simulink model "integracion_ikine"  (R2023b)
settings: Solver=FixedStepDiscrete  StartTime=0.0  StopTime=inf  RelTol=1e-3  EnableMultiTasking=on
undefined symbols (not defined in the file): LF
libraries: instrumentseriallib x3, svdutilitieslib x1, dspnetwork x1
settings Model: SimulationMode=accelerator  Creator=gianm  LastModifiedBy=gianm
settings DebuggingCC: ParameterPrecisionLossMsg=none

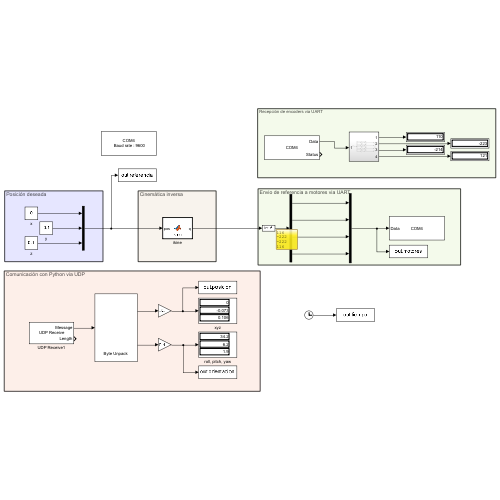
[thumbnail: Simulink's stored preview of the top-level diagram]
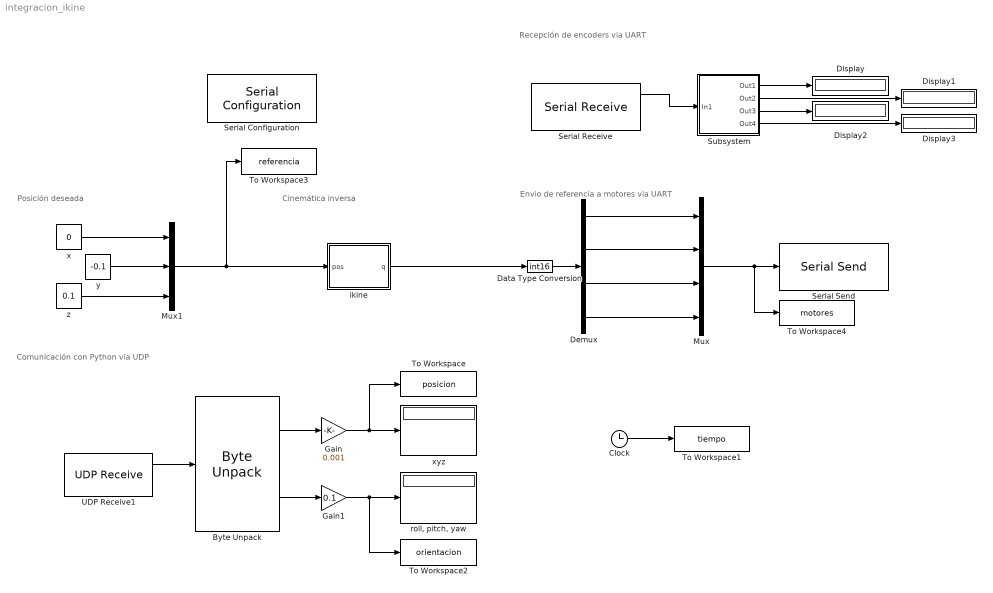
== system integracion_ikine ==
  note: Recepción de encoders via UART
  note: Cinemática inversa
  note: Envio de referencia a motores via UART
  note: Posición deseada
  note: Comunicación con Python via UDP
  Byte Unpack : svdutilitieslib/Byte Unpack  dimensions={[3,1], [3,1]}  datatypes={'int16', 'int16'}  byteAlign=1  blockPlatform=arduinoert
  Clock : Clock
  Data Type Conversion : DataTypeConversion  OutDataTypeStr=int16  SaturateOnIntegerOverflow=off  RndMeth=Floor
  Demux : Demux
  Display{,1..3} (4 alike) : Display
      settings: Format=decimal (Stored Integer)
  Gain : Gain  Gain=0.001
  Gain1 : Gain  Gain=0.1
  Mux : Mux
  Mux1 : Mux  Inputs=3
  Serial Configuration : instrumentseriallib/Serial Configuration  Priority=-200000  PortSel=COM4  Port=COM4  ComPort=COM4  BaudRate=9600  DataBits=8  Parity=none  StopBits=1  ByteOrder=little-endian  FlowControl=none  Timeout=20  SimulateUsing=Interpreted execution  BlockInModel=on  aMode=1
  Serial Receive : instrumentseriallib/Serial Receive  Priority=1  PortSel=COM4  Port=COM4  ComPort=COM4  DataType=uint8  SaveDataType=uint8  ToggleHeader=on  Header=[82]  DataSize=8  ToggleTerminator=on  Terminator=LF ('\n')  CustomTerminator=[]  InputFormat=Column major  ToggleDataSize=on  EnableBlockingMode=off  ActionDataUnavailable=Output last received value  ActionWhenDataUnavailable=Output last received value  CustomValue=0  SampleTime=0.02  SimulateUsing=Interpreted execution  BlockInModel=on  aMode=1
  Serial Send : instrumentseriallib/Serial Send  Priority=1  PortSel=COM4  Port=COM4  ComPort=COM4  Header=[72]  Terminator=LF ('\n')  CustomTerminator=[]  EnableBlockingMode=off  SimulateUsing=Interpreted execution  BlockInModel=on  aMode=1
  Subsystem : Subsystem
  To Workspace : ToWorkspace  VariableName=posicion  SampleTime=0.02
  To Workspace1 : ToWorkspace  VariableName=tiempo  SampleTime=-1
      settings: Save2DSignal=2-D array (concatenate along first dimension)
  To Workspace2 : ToWorkspace  VariableName=orientacion  SampleTime=0.02
  To Workspace3 : ToWorkspace  VariableName=referencia  SampleTime=0.02
      settings: Save2DSignal=2-D array (concatenate along first dimension)
  To Workspace4 : ToWorkspace  VariableName=motores  SampleTime=-1
      settings: Save2DSignal=2-D array (concatenate along first dimension)
  UDP Receive1 : dspnetwork/UDP Receive  localURL='0.0.0.0'  localPort=5005  remoteURL='127.0.0.1'  remotePort=-1  recvBufferSize=16  dims=12  signalDatatype=uint8  isComplex=off  isVarSize=off  showBlockingTime=off  blockingTime=0  sampletime=0.02  blockPlatform=[]
      settings: LibrarySourceBlock=dspsrcs4/UDP Receive
  ikine : MATLAB Function  TreatAsAtomicUnit=on
  "roll, pitch, yaw" : Display
  x : Constant  Value=0
  xyz : Display
  y : Constant  Value=-0.1
  z : Constant  Value=0.1
  wires:
  Serial Receive/1 -> Subsystem/1(In1)
  Mux/1 -> To Workspace4/1, Serial Send/1
  Demux/1 -> Mux/1
  Subsystem/1(Out1) -> Display/1
  Subsystem/4(Out4) -> Display3/1
  Subsystem/3(Out3) -> Display2/1
  Subsystem/2(Out2) -> Display1/1
  Demux/2 -> Mux/2
  Demux/3 -> Mux/3
  Demux/4 -> Mux/4
  x/1 -> Mux1/1
  y/1 -> Mux1/2
  z/1 -> Mux1/3
  ikine/1(q) -> Data Type Conversion/1
  Data Type Conversion/1 -> Demux/1
  Byte Unpack/2 -> Gain1/1
  Byte Unpack/1 -> Gain/1
  UDP Receive1/1 -> Byte Unpack/1
  Mux1/1 -> To Workspace3/1, ikine/1(pos)
  Gain/1 -> To Workspace/1, xyz/1
  Gain1/1 -> To Workspace2/1, "roll, pitch, yaw"/1
  Clock/1 -> To Workspace1/1

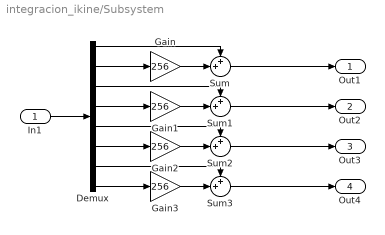
== system integracion_ikine/Subsystem ==
  In1 : Inport
  Demux : Demux  Outputs=8
  Gain{,1..3} (4 alike) : Gain  Gain=256
  Sum{,1..3} (4 alike) : Sum  Inputs=++|  OutDataTypeStr=int16
  Out1 : Outport
  Out2 : Outport  Port=2
  Out3 : Outport  Port=3
  Out4 : Outport  Port=4
  wires:
  In1/1 -> Demux/1
  Demux/2 -> Gain/1
  Gain/1 -> Sum/2
  Demux/1 -> Sum/1
  Sum/1 -> Out1/1
  Demux/4 -> Gain1/1
  Demux/3 -> Sum1/1
  Gain1/1 -> Sum1/2
  Demux/6 -> Gain2/1
  Sum2/1 -> Out3/1
  Demux/5 -> Sum2/1
  Gain2/1 -> Sum2/2
  Demux/8 -> Gain3/1
  Demux/7 -> Sum3/1
  Gain3/1 -> Sum3/2
  Sum1/1 -> Out2/1
  Sum3/1 -> Out4/1

== matlab function integracion_ikine/ikine ==
  data: pos input; q output
function q = ikine(pos)

R = eye(3);
% ikine- Cinemática inversa
%
% Inputs:
%   pos     -> [x; y; z] posición del centro del efector (3x1)
%   R       -> orientación del efector (3x3)
% Output:
%   q -> vector [4x1] con giro de los motores

% Posición y orientación inicial 
initial_pos = [0; 0; 0.053];
initial_R = eye(3);

% Anclajes de la base (4 esquinas)
anchors = [-0.27/2  -0.27/2  0.27/2  0.27/2;
            0.27/2  -0.27/2 -0.27/2  0.27/2;
            0.22  0.22  0.22  0.22]; % (3x4)

% Offsets desde el centro del efector hasta cada esquina
% prisma de 0.1 x 0.1 x 0.030
Lx = 0.1; Ly = 0.1; Lz = 0.0;
offsets = [ -Lx  -Lx  Lx  Lx;
             Ly  -Ly -Ly  Ly;
             Lz  Lz  Lz  Lz ]/2; % (3x4)

% Longitud actual del cable
L = zeros(4,1);

% Longitud inicial del cable
L0 = zeros(4,1);

for i = 1:4
    % Posición del punto de conexión en el efector
    P = pos + R * offsets(:,i);
    initial_P = initial_pos + initial_R * offsets(:,i);
    
    % Longitud del cable i
    L(i) = norm(P - anchors(:,i));
    L0(i) = norm(initial_P - anchors(:,i));
end

% Giro del motor
R_carrete = 0.03/2;
q = (L - L0) / R_carrete; % rad
q = q * 180 / pi; % deg

% Si q es +, el motor gira en sentido antihorario (soltar cable)
% Si q es -, el motor gira en sentido horario (retraer cable)

end
